simulink model "controller_unit_integration_tests_final"  (R2024a)
settings: Solver=FixedStepAuto  StartTime=0.0  StopTime=500  RelTol=1e-3
libraries: simulink x6
settings Model: Creator=mahdy  LastModifiedBy=mahdy

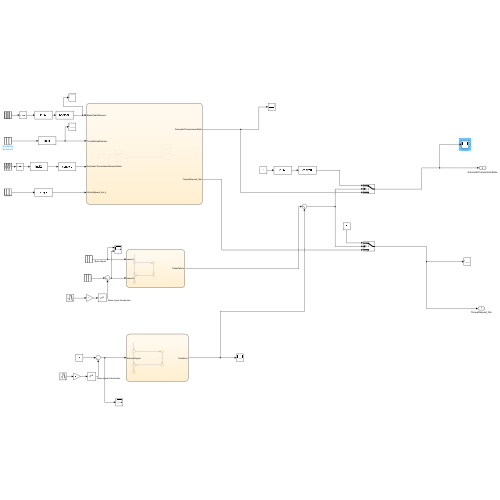
[thumbnail: Simulink's stored preview of the top-level diagram]
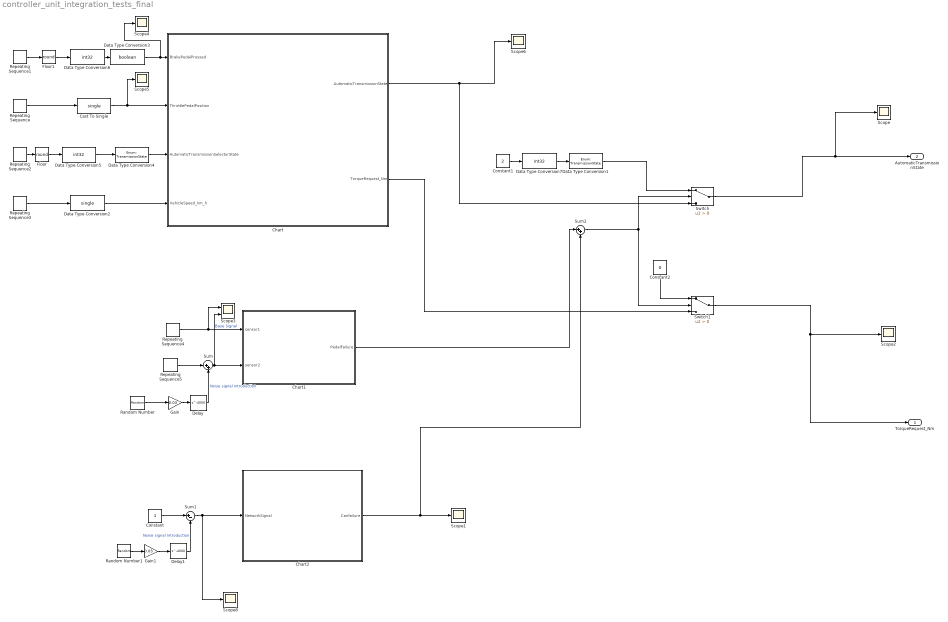
== system controller_unit_integration_tests_final ==
  Cast To Single : DataTypeConversion  OutDataTypeStr=single  SaturateOnIntegerOverflow=off  RndMeth=Floor
  Chart : Stateflow chart  TreatAsAtomicUnit=on
  Chart1 : Stateflow chart  TreatAsAtomicUnit=on
  Chart2 : Stateflow chart  TreatAsAtomicUnit=on
  Constant : Constant
  Constant1 : Constant  Value=2
  Constant2 : Constant  Value=0
  Data Type Conversion1 : DataTypeConversion  OutDataTypeStr=Enum: TransmissionState  SaturateOnIntegerOverflow=off  RndMeth=Floor  LockScale=on
  Data Type Conversion2 : DataTypeConversion  OutDataTypeStr=single  SaturateOnIntegerOverflow=off  RndMeth=Floor
  Data Type Conversion3 : DataTypeConversion  OutDataTypeStr=boolean  SaturateOnIntegerOverflow=off  RndMeth=Floor  LockScale=on
  Data Type Conversion4 : DataTypeConversion  OutDataTypeStr=Enum: TransmissionState  SaturateOnIntegerOverflow=off  RndMeth=Floor  LockScale=on
  Data Type Conversion5 : DataTypeConversion  OutDataTypeStr=int32  SaturateOnIntegerOverflow=off  RndMeth=Floor  LockScale=on
  Data Type Conversion6 : DataTypeConversion  OutDataTypeStr=int32  SaturateOnIntegerOverflow=off  RndMeth=Floor  LockScale=on
  Data Type Conversion7 : DataTypeConversion  OutDataTypeStr=int32  SaturateOnIntegerOverflow=off  RndMeth=Floor  LockScale=on
  Delay : Delay  DelayLength=4000  SampleTime=0.1
  Delay1 : Delay  DelayLength=4000  SampleTime=0.1
  Floor : Rounding  Operator=round
  Floor1 : Rounding  Operator=round
  Gain : Gain  Gain=0.03
  Gain1 : Gain  Gain=0.03
  Random Number : RandomNumber  SampleTime=0.1
  Random Number1 : RandomNumber  Mean=4  SampleTime=0.1
  Repeating Sequence : simulink/Sources/Repeating Sequence  rep_seq_t=[0 3.9 4 500]  rep_seq_y=[0 0 1 1]
  Repeating Sequence1 : simulink/Sources/Repeating Sequence  rep_seq_t=[0 2.999 3 49.9 80.0 82.0 92.1 500]  rep_seq_y=[1 1 0 0 1 1 0 0]
  Repeating Sequence2 : simulink/Sources/Repeating Sequence  rep_seq_t=[0 1.999 2 10 79.9 80.0 500]  rep_seq_y=[0 0 4 4 4 1 4]
  Repeating Sequence3 : simulink/Sources/Repeating Sequence  rep_seq_t=[0 3.9 4 29.9 30 39.9 40 82.9 83 500]  rep_seq_y=[0 0 90 90 60 60 0 0 -20 -20]
  Repeating Sequence4 : simulink/Sources/Repeating Sequence  rep_seq_t=[0 3.9 4 500]  rep_seq_y=[0 0 1 1]
  Repeating Sequence5 : simulink/Sources/Repeating Sequence  rep_seq_t=[0 3.9 4 500]  rep_seq_y=[0 0 1 1]
  Scope{,1..2,4..6,8} (7 alike) : Scope
  Scope3 : Scope  NumInputPorts=2
  Sum : Sum  Inputs=|++
  Sum1 : Sum  Inputs=|+-
  Sum2 : Sum  Inputs=|++
  Switch : Switch  Criteria=u2 > Threshold  SaturateOnIntegerOverflow=off  InputSameDT=off
  Switch1 : Switch  Criteria=u2 > Threshold  SaturateOnIntegerOverflow=off  InputSameDT=off
  TorqueRequest_Nm : Outport  OutDataTypeStr=single  Unit=N*m
  AutomaticTransmissionState : Outport  Port=2  OutDataTypeStr=Enum: TransmissionState
  wires:
  Chart/2(TorqueRequest_Nm) -> Switch1/3
  Repeating Sequence/1 -> Cast To Single/1
  Cast To Single/1 -> Scope5/1, Chart/2(ThrottlePedalPosition)
  Data Type Conversion2/1 -> Chart/4(VehicleSpeed_km_h)
  Repeating Sequence3/1 -> Data Type Conversion2/1
  Chart/1(AutomaticTransmissionState) -> Switch/3, Scope6/1
  Repeating Sequence1/1 -> Floor1/1
  Repeating Sequence2/1 -> Floor/1
  Floor/1 -> Data Type Conversion5/1
  Floor1/1 -> Data Type Conversion6/1
  Data Type Conversion5/1 -> Data Type Conversion4/1
  Data Type Conversion6/1 -> Data Type Conversion3/1
  Data Type Conversion3/1 -> Scope4/1, Chart/1(BrakePedalPressed)
  Data Type Conversion4/1 -> Chart/3(AutomaticTransmissionSelectorState)
  Repeating Sequence5/1 -> Sum/1
  Random Number/1 -> Gain/1
  Sum/1 -> Scope3/2, Chart1/2(sensor2)
  Gain/1 -> Delay/1
  Delay/1 -> Sum/2  "Noise signal Introduction"
  Repeating Sequence4/1 -> Scope3/1, Chart1/1(sensor1)  "Base Signal"
  Chart1/1(PedalFailure) -> Sum2/1
  Random Number1/1 -> Gain1/1
  Constant/1 -> Sum1/1
  Gain1/1 -> Delay1/1
  Delay1/1 -> Sum1/2  "Noise signal Introduction"
  Sum1/1 -> Scope8/1, Chart2/1(NetworkSignal)
  Chart2/1(Canfailure) -> Sum2/2, Scope1/1
  Constant1/1 -> Data Type Conversion7/1
  Data Type Conversion1/1 -> Switch/1
  Data Type Conversion7/1 -> Data Type Conversion1/1
  Sum2/1 -> Switch/2, Switch1/2
  Switch/1 -> Scope/1, AutomaticTransmissionState/1
  Constant2/1 -> Switch1/1
  Switch1/1 -> TorqueRequest_Nm/1, Scope2/1

== stateflow chart controller_unit_integration_tests_final/Chart ==
  state Reverse
    entry:
    AutomaticTransmissionState =TransmissionState. Reverse;
    during:
    TorqueRequest_Nm = -ThrottlePedalPosition*MAX_TORQUE_REVERSE;
  state Park
    entry:
    AutomaticTransmissionState = TransmissionState.Park;
    TorqueRequest_Nm = 0;
  state Neutral
    entry:
    AutomaticTransmissionState = TransmissionState.Neutral;
    TorqueRequest_Nm = 0;
  state Bmode
    entry:
    AutomaticTransmissionState = TransmissionState.Brake;
    state Acceleration
      during:
      TorqueRequest_Nm =MAX_TORQUE*(ThrottlePedalPosition-1/3)*3/2;
    state Regenerative_Braking
      during:
      TorqueRequest_Nm =- MAX_TORQUE*(1-3*ThrottlePedalPosition)
    state Stop
      entry:
      TorqueRequest_Nm = 0;
    (default) -> Acceleration
    Acceleration -> Regenerative_Braking : [ThrottlePedalPosition<=1/3]
    Regenerative_Braking -> Acceleration [order 1] : [ThrottlePedalPosition>1/3]
    Stop -> Acceleration : [ThrottlePedalPosition>1/3]
    Regenerative_Braking -> Stop [order 2] : [ 0<ThrottlePedalPosition<=1/3 &&VehicleSpeed_km_h<=0.05 ]
  state Drive
    entry:
    AutomaticTransmissionState = TransmissionState.Drive;
    during:
    TorqueRequest_Nm = ThrottlePedalPosition*MAX_TORQUE;
  Reverse -> Neutral : [AutomaticTransmissionSelectorState ==TransmissionState. Neutral || AutomaticTransmissionSelectorState ==TransmissionState. Drive ||AutomaticTransmissionSelectorState ==TransmissionState. Brake||AutomaticTransmissionSelectorState ==TransmissionState. Park]
  Neutral -> Reverse [order 3] : [ VehicleSpeed_km_h<5 && AutomaticTransmissionSelectorState ==TransmissionState. Reverse &&BrakePedalPressed ==1]
  (default) -> Park
  Neutral -> Park [order 2] : [BrakePedalPressed ==1 && abs(VehicleSpeed_km_h)<5 && AutomaticTransmissionSelectorState == TransmissionState.Park]
  Park -> Neutral : [BrakePedalPressed ==1 && (AutomaticTransmissionSelectorState == TransmissionState.Reverse||AutomaticTransmissionSelectorState == TransmissionState.Neutral || AutomaticTransmissionSelectorState==TransmissionState.Brake|| AutomaticTransmissionSelectorState == TransmissionState.Drive)]
  Drive -> Neutral [order 1] : [AutomaticTransmissionSelectorState ==TransmissionState. Neutral||AutomaticTransmissionSelectorState == TransmissionState.Reverse||AutomaticTransmissionSelectorState == TransmissionState.Park]
  Neutral -> Drive [order 1] : [BrakePedalPressed==1 && VehicleSpeed_km_h>-5 && AutomaticTransmissionSelectorState ==TransmissionState. Drive || AutomaticTransmissionSelectorState == TransmissionState.Brake ]
  Drive -> Bmode [order 2] : [AutomaticTransmissionSelectorState == TransmissionState.Brake ]
  Bmode -> Drive : [AutomaticTransmissionSelectorState == TransmissionState.Drive||AutomaticTransmissionSelectorState == TransmissionState.Neutral||AutomaticTransmissionSelectorState == TransmissionState.Reverse||AutomaticTransmissionSelectorState == TransmissionState.Park]
  data: BrakePedalPressed input boolean; ThrottlePedalPosition input single; AutomaticTransmissionSelectorState input Enum: TransmissionState; VehicleSpeed_km_h input single; AutomaticTransmissionState output Enum: TransmissionState; TorqueRequest_Nm output single; MAX_TORQUE_REVERSE local =40; MAX_TORQUE local =80

== stateflow chart controller_unit_integration_tests_final/Chart1 ==
  (default) -> (junction 22) : % PedalSensorFailure
  (junction 22) -> (junction 23) [order 1] : [sensor1-sensor2>=0.05|| error == 1]
  (junction 22) -> (junction 24) [order 2] : {PedalFailure=0;error = 0}
  (junction 23) -> (junction 25) : {PedalFailure=1;error=1}
  (junction 25) -> (junction 24)
  (junction 24) -> (junction 26)
  data: sensor1 input; sensor2 input; PedalFailure output; error local =0

== stateflow chart controller_unit_integration_tests_final/Chart2 ==
  (default) -> (junction 20) : % CanNetworkTest
  (junction 20) -> (junction 21) [order 1] : [NetworkSignal<1||error ==1]
  (junction 20) -> (junction 22) [order 2] : {Canfailure=0;error = 0}
  (junction 21) -> (junction 23) : {Canfailure=1;error = 1}
  (junction 23) -> (junction 22)
  (junction 22) -> (junction 24)
  data: NetworkSignal input; Canfailure output; error local =0
